simulink model "Problem2"  (R2020a)
settings: Solver=VariableStepAuto  StartTime=0.0  StopTime=10.0  RelTol=1e-3
undefined symbols (not defined in the file): be, bv, Ie, Iv
settings Model: Creator=tanu  LastModifiedBy=tanu

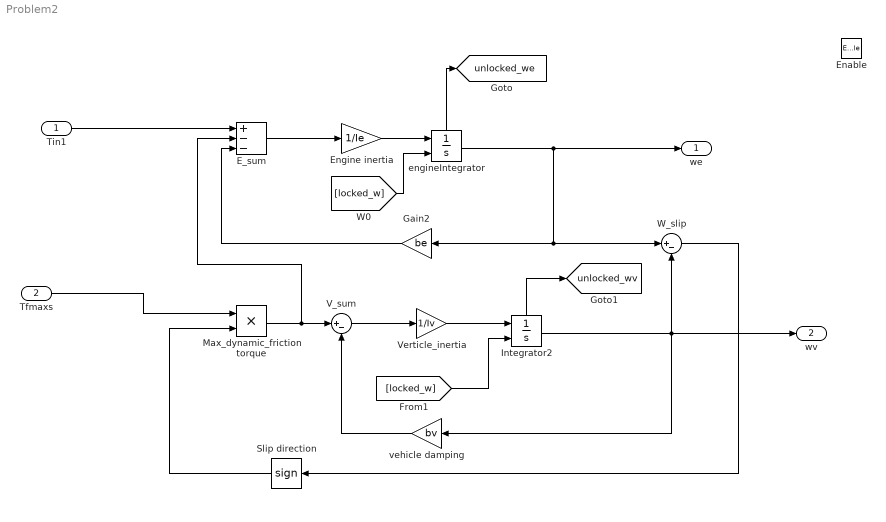
== system Problem2 ==
  Tin1 : Inport
  Tfmaxs : Inport  Port=2
  Enable : EnablePort
  E_sum : Sum  Inputs=+--
  Engine inertia : Gain  Gain=1/Ie
  Gain2 : Gain  Gain=be
  Integrator2 : Integrator  InitialConditionSource=external  ShowStatePort=on
  Max_dynamic_friction torque : Product
  Slip direction : Signum
  V_sum : Sum  Inputs=|+-
  Verticle_inertia : Gain  Gain=1/Iv
  W_slip : Sum  Inputs=|+-
  engineIntegrator : Integrator  InitialConditionSource=external  ShowStatePort=on
  vehicle damping : Gain  Gain=bv
  we : Outport
  wv : Outport  Port=2
  tag scope: unlocked_we=global, unlocked_wv=global
  wires:
  engineIntegrator/1 -> we/1, Gain2/1, W_slip/1
  Verticle_inertia/1 -> Integrator2/1
  E_sum/1 -> Engine inertia/1
  Tfmaxs/1 -> Max_dynamic_friction torque/1
  engineIntegrator/State -> [unlocked_we]
  [locked_w] -> Integrator2/2
  Integrator2/1 -> wv/1, vehicle damping/1, W_slip/2
  Tin1/1 -> E_sum/1
  Slip direction/1 -> Max_dynamic_friction torque/2
  Integrator2/State -> [unlocked_wv]
  vehicle damping/1 -> V_sum/2
  W_slip/1 -> Slip direction/1
  Gain2/1 -> E_sum/3
  [locked_w] -> engineIntegrator/2
  Max_dynamic_friction torque/1 -> V_sum/1, E_sum/2
  Engine inertia/1 -> engineIntegrator/1
  V_sum/1 -> Verticle_inertia/1
